simulink model "RW_Time_Delay_Analysis_mdl"  (R2025b)
settings: Solver=VariableStepAuto  StartTime=0.0  StopTime=10.0  RelTol=1e-3
values from neighbouring files (symbols this model uses):
  Kd = 0.95    [RW_Time_Delay_Analysis.m]    (also in RW_Time_Delay_Analysis_Simulink_Params.m; RW_Time_Delay_Analysis_new_implementation.m)
  Ki = 0.1    [RW_Time_Delay_Analysis.m]    (also in RW_Time_Delay_Analysis_Simulink_Params.m; RW_Time_Delay_Analysis_new_implementation.m)
  Kp = 0.8    [RW_Time_Delay_Analysis.m]    (also in RW_Time_Delay_Analysis_Simulink_Params.m; RW_Time_Delay_Analysis_new_implementation.m)
  Ts = 0.1    [RW_Time_Delay_Analysis.m]    (also in RW_Time_Delay_Analysis_Simulink_Params.m; RW_Time_Delay_Analysis_new_implementation.m; RW_Time_Delay_PID_Tuner.m; RW_Time_Delay_PID_Tuner_Script.m)
undefined symbols (not defined in the file or in its folder): DiscIntNeverNeededParam, dspblkCoreblockFVToolHelper, gcbh
libraries: discretizing x4
settings Model: Creator=barinmoghimi  LastModifiedBy=barinmoghimi

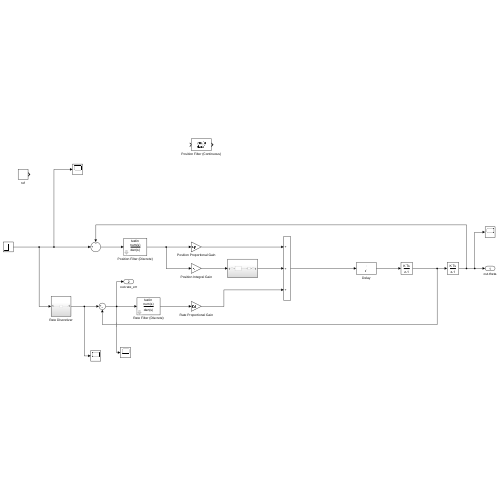
[thumbnail: Simulink's stored preview of the top-level diagram]
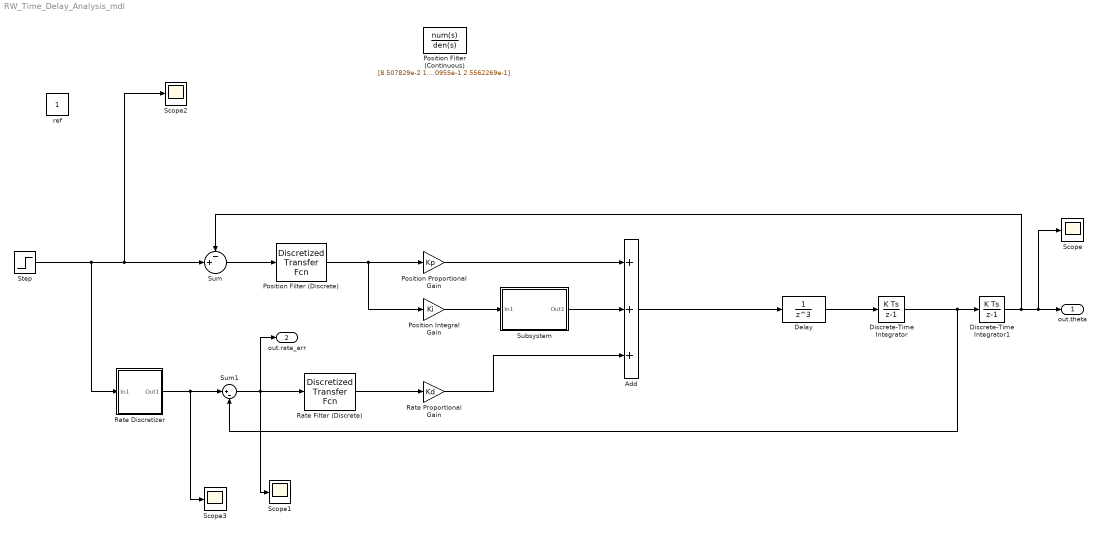
== system RW_Time_Delay_Analysis_mdl ==
  Add : Sum  Inputs=+++
  Delay : DiscreteTransferFcn  LoadFcn=dspblkCoreblockFVToolHelper(gcbh,'load');  Denominator=[1 0 0 0]
      settings: CopyFcn=dspblkCoreblockFVToolHelper(gcbh,'copy');  DeleteFcn=dspblkCoreblockFVToolHelper(gcbh,'close');  ModelCloseFcn=dspblkCoreblockFVToolHelper(gcbh,'close');  PreSaveFcn=dspblkCoreblockFVToolHelper(gcbh,'presave');  PostSaveFcn=dspblkCoreblockFVToolHelper(gcbh,'postsave');  CloseFcn=dspblkCoreblockFVToolHelper(gcbh,'close');
  Discrete-Time Integrator : DiscreteIntegrator  SampleTime=Ts  ICPrevOutput=DiscIntNeverNeededParam  ICPrevScaledInput=DiscIntNeverNeededParam
  Discrete-Time Integrator1 : DiscreteIntegrator  SampleTime=Ts  ICPrevOutput=DiscIntNeverNeededParam  ICPrevScaledInput=DiscIntNeverNeededParam
  Position Filter (Continuous) : TransferFcn  Numerator=[8.507829e-2 1.7015657e-1 8.50782e-2]  Denominator=[1.0e+0 -9.1530955e-1 2.5562269e-1]
  Position Filter (Discrete) : discretizing/Discretized Transfer Fcn  Numerator=[8.507829e-2 1.7015657e-1 8.50782e-2]  Denominator=[1.0e+0 -9.1530955e-1 2.5562269e-1]  AbsTol=auto  SampleTime=1  method=tustin  Wc=1
  Position Integral Gain : Gain  Gain=Ki
  Position Proportional Gain : Gain  Gain=Kp
  Rate Discretizer : Subsystem
  Rate Filter (Discrete) : discretizing/Discretized Transfer Fcn  Numerator=[8.507829e-2 1.7015657e-1 8.50782e-2]  Denominator=[1.0e+0 -9.1530955e-1 2.5562269e-1]  AbsTol=auto  SampleTime=1  method=tustin  Wc=1
  Rate Proportional Gain : Gain  Gain=Kd
  Scope{,1..3} (4 alike) : Scope
      Scope settings: ActiveDisplayYMinimum=-1  ActiveDisplayYMaximum=1
      Scope1 settings: ActiveDisplayYMinimum=-1  ActiveDisplayYMaximum=1
      Scope2 settings: ActiveDisplayYMinimum=-1  ActiveDisplayYMaximum=1  DataLoggingVariableName=ScopeData2
      Scope3 settings: ActiveDisplayYMinimum=-2.5  ActiveDisplayYMaximum=2.5  DataLoggingVariableName=ScopeData3
  Step : Step  SampleTime=0
  Subsystem : Subsystem
  Sum : Sum  Inputs=-+|
  Sum1 : Sum  Inputs=|+-
  ref : Constant
  out.theta : Outport
  out.rate_err : Outport  Port=2
  wires:
  Rate Discretizer/1(Out1) -> Scope3/1, Sum1/1
  Sum1/1 -> Scope1/1, Rate Filter (Discrete)/1, out.rate_err/1
  Rate Filter (Discrete)/1 -> Rate Proportional Gain/1
  Rate Proportional Gain/1 -> Add/3
  Position Proportional Gain/1 -> Add/1
  Add/1 -> Delay/1
  Delay/1 -> Discrete-Time Integrator/1
  Discrete-Time Integrator1/1 -> Sum/1, Scope/1, out.theta/1
  Position Filter (Discrete)/1 -> Position Proportional Gain/1, Position Integral Gain/1
  Sum/1 -> Position Filter (Discrete)/1
  Subsystem/1(Out1) -> Add/2
  Position Integral Gain/1 -> Subsystem/1(In1)
  Discrete-Time Integrator/1 -> Sum1/2, Discrete-Time Integrator1/1
  Step/1 -> Rate Discretizer/1(In1), Scope2/1, Sum/2

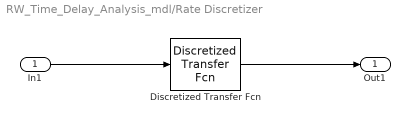
== system RW_Time_Delay_Analysis_mdl/Rate Discretizer ==
  In1 : Inport
  Discretized Transfer Fcn : discretizing/Discretized Transfer Fcn  Numerator=[1 0]  Denominator=[1]  AbsTol=auto  SampleTime=1  method=tustin  Wc=1
  Out1 : Outport
  wires:
  Discretized Transfer Fcn/1 -> Out1/1
  In1/1 -> Discretized Transfer Fcn/1

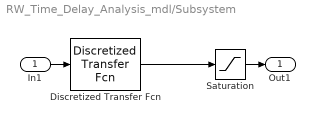
== system RW_Time_Delay_Analysis_mdl/Subsystem ==
  In1 : Inport
  Discretized Transfer Fcn : discretizing/Discretized Transfer Fcn  Numerator=[1]  Denominator=[1 0]  AbsTol=auto  SampleTime=Ts  method=tustin  Wc=1
  Saturation : Saturate  UpperLimit=pi  LowerLimit=-pi
  Out1 : Outport
  wires:
  Discretized Transfer Fcn/1 -> Saturation/1
  Saturation/1 -> Out1/1
  In1/1 -> Discretized Transfer Fcn/1
